simulink model "PiRegler"  (R2025b)
settings: Solver=FixedStepAuto  StartTime=0.0  StopTime=2  FixedStep=.001  RelTol=1e-3  EnableMultiTasking=on
PostLoadFcn:
  | PostLoadFcn
values from neighbouring files (symbols this model uses):
  A1 = -1.9425    [Plant_Parameter.mat]
  A2 = 0.9425    [Plant_Parameter.mat]
  B0 = 0    [Plant_Parameter.mat]
  B1 = 0.001    [Plant_Parameter.mat]
  B2 = 0.001    [Plant_Parameter.mat]
  I_Gain = -0.03    [Regler_Parameter.mat]
  I_InErrMap = [-1 -0.5 -0.25 -0.05 0 0.05 0.25 0.5 1]    [Regler_Parameter.mat]
  I_OutMap = [1 0.75 0.6 0 0 0 0.6 0.75 1]    [Regler_Parameter.mat]
  P_Gain = 0.74    [Regler_Parameter.mat]
  P_InErrMap = [-1 -0.25 -0.01 0 0.01 0.25 1]    [Regler_Parameter.mat]
  P_OutMap = [1 0.25 0 0 0 0.25 1]    [Regler_Parameter.mat]
undefined symbols (not defined in the file or in its folder): DiscIntNeverNeededParam
settings Model: ExtModeAutoUpdateStatusClock=off  Creator=The MathWorks Inc.  LastModifiedBy=danieltchoudovski
settings SolverCC: AlgebraicLoopSolver=TrustRegion
settings DataIOCC: LimitDataPoints=on  SaveFormat=Array  SignalLoggingSaveFormat=ModelDataLogs  SaveOutput=off  SaveTime=off
settings OptimizationCC: BlockReduction=off  OptimizeBlockIOStorage=off  ExpressionDepthLimit=2147483647.0  InitFltsAndDblsToZero=on  LifeSpan=inf  OptimizeDataStoreBuffers=off  BusAssignmentInplaceUpdate=off
settings DebuggingCC: UnderspecifiedInitializationDetection=Classic  SignalResolutionControl=TryResolveAllWithWarning  SolverPrmCheckMsg=warning  MultiTaskRateTransMsg=warning  UnconnectedInputMsg=warning  UnconnectedOutputMsg=warning  UnconnectedLineMsg=warning  AllowSymbolicDim=off  StateNameClashWarn=warning  SFUnexpectedBacktrackingDiag=warning  SFNoUnconditionalDefaultTransitionDiag=warning  SFExecutionAtInitializationDiag=none  ArithmeticOperatorsInVariantConditions=warning
settings HardwareCC: ProdBitPerPointer=32.0  ProdBitPerSizeT=32.0  ProdBitPerPtrDiffT=32.0  ProdLargestAtomicFloat=None  ProdIntDivRoundTo=Undefined  ProdEndianess=Unspecified  ProdWordSize=32.0  ProdHWDeviceType=Generic->32-bit Embedded Processor
settings ModelReferenceCC: EnableRefExpFcnMdlSchedulingChecks=on  ModelReferenceNumInstancesAllowed=Single  PropagateSignalLabelsOutOfModel=off
settings SFSimCC: SimUseLocalCustomCode=off  CustomCodeUndefinedFunction=UseInterfaceOnly
settings RTWCC: GenCodeOnly=on  GenerateReport=on  RTWUseLocalCustomCode=off  BuildConfiguration=Debug  LaunchReport=on  GPUComputeCapability=3.5
settings CodeAppCC: ForceParamTrailComments=on  MATLABSourceComments=on  EnableCustomComments=on
settings GRTTargetCC: MultiInstanceErrorCode=Warning  TargetLangStandard=C89/C90 (ANSI)  CombineSignalStateStructs=on  SubcomponentCodeInterfacePackaging=Nonreusable function  SupportVariableSizeSignals=on
settings ConfigComp: CovMetricSettings=dw  CovSaveCumulativeToWorkspaceVar=on  CovSaveSingleToWorkspaceVar=on  CovExternalEMLEnable=off  CovSFcnEnable=off

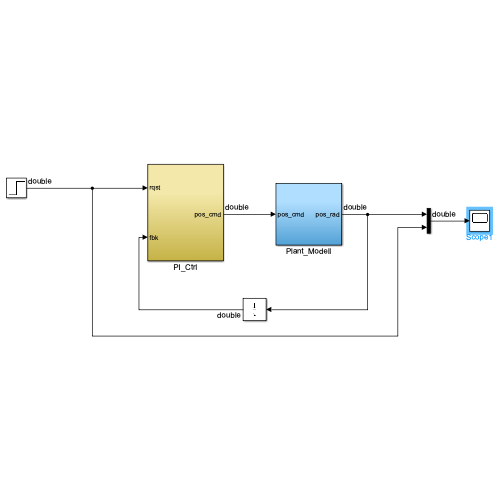
[thumbnail: Simulink's stored preview of the top-level diagram]
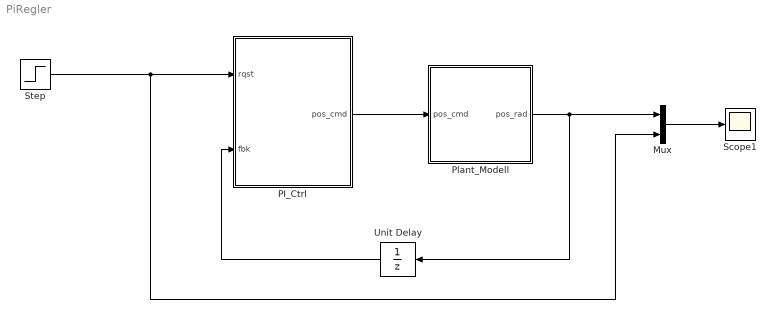
== system PiRegler ==
  Mux : Mux  Inputs=2
  PI_Ctrl : Subsystem
      settings: RTWFileNameOpts=Use function name
  Plant_Modell : Subsystem
  Scope1 : Scope
      settings: ActiveDisplayYMinimum=-0.14883425599527916  ActiveDisplayYMaximum=1.3395083039575126  DataLoggingSaveFormat=Array
  Step : Step  SampleTime=0
  Unit Delay : UnitDelay  SampleTime=-1  HasFrameUpgradeWarning=on
  wires:
  PI_Ctrl/1(pos_cmd) -> Plant_Modell/1(pos_cmd)
  Plant_Modell/1(pos_rad) -> Mux/1, Unit Delay/1
  Step/1 -> Mux/2, PI_Ctrl/1(rqst)
  Mux/1 -> Scope1/1
  Unit Delay/1 -> PI_Ctrl/2(fbk)

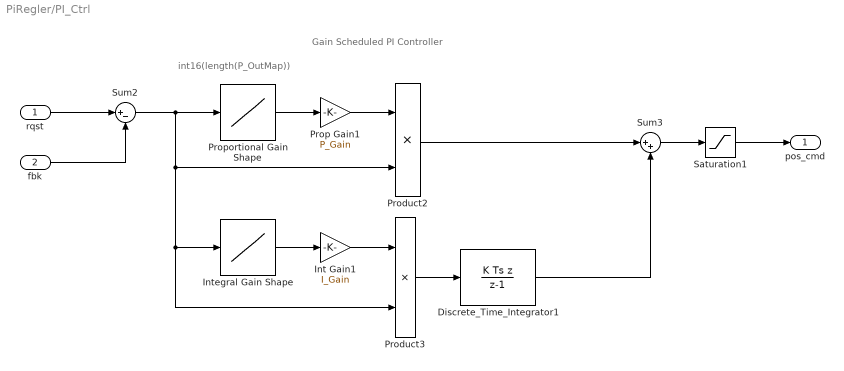
== system PiRegler/PI_Ctrl ==
  note: Gain Scheduled PI Controller
  note: int16(length(P_OutMap))
  rqst : Inport
  fbk : Inport  Port=2
  Discrete_Time_Integrator1 : DiscreteIntegrator  IntegratorMethod=Integration: Backward Euler  SampleTime=-1  OutDataTypeStr=Inherit: Inherit via back propagation  UpperSaturationLimit=1  LowerSaturationLimit=-1  ICPrevOutput=DiscIntNeverNeededParam  ICPrevScaledInput=DiscIntNeverNeededParam
  Int Gain1 : Gain  Gain=I_Gain  OutDataTypeStr=Inherit: Same as input  ParamDataTypeStr=Inherit: Same as input
      settings: AttributesFormatString=%<Gain>
  Integral Gain Shape : Lookup_n-D  NumberOfTableDimensions=1  BreakpointsForDimension1=I_InErrMap  Table=I_OutMap  ExtrapMethod=Clip  InternalRulePriority=Speed
  Product2 : Product  RndMeth=Zero
  Product3 : Product  RndMeth=Zero
  Prop Gain1 : Gain  Gain=P_Gain  OutDataTypeStr=Inherit: Same as input  ParamDataTypeStr=Inherit: Same as input
      settings: AttributesFormatString=%<Gain>
  Proportional Gain Shape : Lookup_n-D  NumberOfTableDimensions=1  BreakpointsForDimension1=P_InErrMap  Table=P_OutMap  ExtrapMethod=Clip  InternalRulePriority=Speed
  Saturation1 : Saturate  UpperLimit=1  LowerLimit=-1  OutDataTypeStr=Inherit: Inherit via back propagation
  Sum2 : Sum  Inputs=|+-  InputSameDT=on
  Sum3 : Sum  Inputs=|++  InputSameDT=on
  pos_cmd : Outport  VectorParamsAs1DForOutWhenUnconnected=off
  wires:
  Product2/1 -> Sum3/1
  Prop Gain1/1 -> Product2/1
  Product3/1 -> Discrete_Time_Integrator1/1
  Int Gain1/1 -> Product3/1
  Proportional Gain Shape/1 -> Prop Gain1/1
  Integral Gain Shape/1 -> Int Gain1/1
  Sum2/1 -> Product3/2, Integral Gain Shape/1, Product2/2, Proportional Gain Shape/1
  fbk/1 -> Sum2/2
  rqst/1 -> Sum2/1
  Saturation1/1 -> pos_cmd/1
  Sum3/1 -> Saturation1/1
  Discrete_Time_Integrator1/1 -> Sum3/2

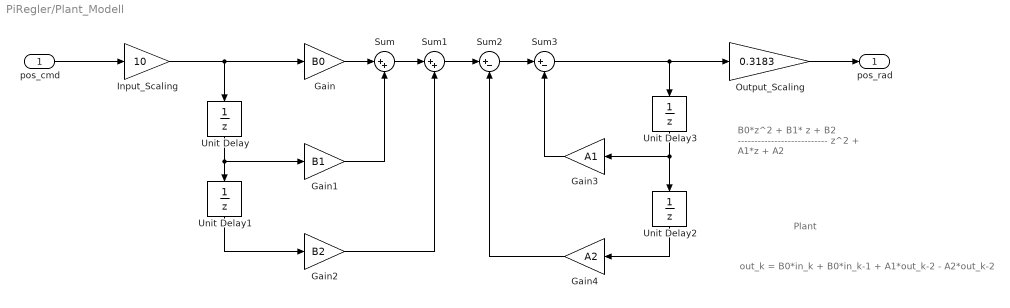
== system PiRegler/Plant_Modell ==
  note: Plant
  note: B0*z^2 + B1* z + B2
      | ---------------------------
      |    z^2 + A1*z + A2
  note: out_k = B0*in_k + B0*in_k-1 + A1*out_k-2 - A2*out_k-2
  pos_cmd : Inport
  Gain : Gain  Gain=B0
  Gain1 : Gain  Gain=B1
  Gain2 : Gain  Gain=B2
  Gain3 : Gain  Gain=A1
  Gain4 : Gain  Gain=A2
  Input_Scaling : Gain  Gain=10
  Output_Scaling : Gain  Gain=0.3183
  Sum : Sum  Inputs=|++
  Sum1 : Sum  Inputs=|++
  Sum2 : Sum  Inputs=|+-
  Sum3 : Sum  Inputs=|+-
  Unit Delay{,1..3} (4 alike) : UnitDelay  SampleTime=-1  HasFrameUpgradeWarning=on
  pos_rad : Outport  VectorParamsAs1DForOutWhenUnconnected=off
  wires:
  pos_cmd/1 -> Input_Scaling/1
  Input_Scaling/1 -> Gain/1, Unit Delay/1
  Output_Scaling/1 -> pos_rad/1
  Unit Delay/1 -> Gain1/1, Unit Delay1/1
  Unit Delay1/1 -> Gain2/1
  Gain/1 -> Sum/1
  Gain1/1 -> Sum/2
  Sum/1 -> Sum1/1
  Gain2/1 -> Sum1/2
  Sum3/1 -> Output_Scaling/1, Unit Delay3/1
  Unit Delay3/1 -> Gain3/1, Unit Delay2/1
  Gain3/1 -> Sum3/2
  Unit Delay2/1 -> Gain4/1
  Gain4/1 -> Sum2/2
  Sum1/1 -> Sum2/1
  Sum2/1 -> Sum3/1
